simulink model "PID_tuningmodel"  (Simulink 8.3)
settings: Solver=ode5  StartTime=0.0  StopTime=.1  FixedStep=1/20000  RelTol=1e-3
PreLoadFcn:
  | Kp =0.7748; Ki =0.2084; Kd =0.9246;
undefined symbols (not defined in the file or in its folder): K, P1, P2, Z1, Z2
settings Model: Creator=e5104961  LastModifiedBy=e5104961
settings DataIOCC: LimitDataPoints=off  SignalLoggingName=sigsOut
settings DebuggingCC: SaveWithParameterizedLinksMsg=none  SignalResolutionControl=TryResolveAllWithWarning  SolverPrmCheckMsg=none  MultiTaskDSMMsg=warning  MultiTaskCondExecSysMsg=none  StateNameClashWarn=none
settings HardwareCC: TargetUnknown=on
settings RTWCC: IncludeERTFirstTime=on

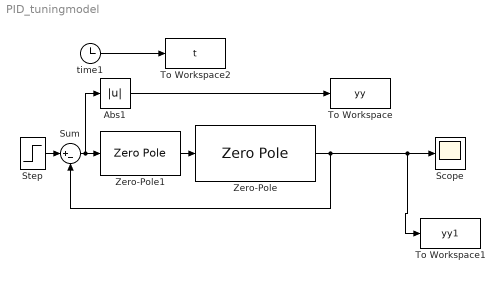
== system PID_tuningmodel ==
  Abs1 : Abs  SaturateOnIntegerOverflow=on
  Scope : Scope
      settings: TimeRange=0.5  YMin=0  YMax=1.2
  Step : Step  Time=0  SampleTime=0
  Sum : Sum  Inputs=|+-  SaturateOnIntegerOverflow=on
  To Workspace : ToWorkspace  VariableName=yy  SampleTime=-1
  To Workspace1 : ToWorkspace  VariableName=yy1  SampleTime=-1
  To Workspace2 : ToWorkspace  VariableName=t  SampleTime=-1
  Zero-Pole : ZeroPole  Zeros=[1200]  Poles=[-389.8 212.5]  Gain=-85
  Zero-Pole1 : ZeroPole  Zeros=[-Z1 -Z2]  Poles=[-P1 -P2]  Gain=[K]
  time1 : Clock
  wires:
  Zero-Pole/1 -> To Workspace1/1, Scope/1, Sum/2
  Step/1 -> Sum/1
  Sum/1 -> Abs1/1, Zero-Pole1/1
  time1/1 -> To Workspace2/1
  Abs1/1 -> To Workspace/1
  Zero-Pole1/1 -> Zero-Pole/1
